simulink model "Buck_converter"  (R2015a)
settings: Solver=ode45  StartTime=0.0  StopTime=1.0  MaxStep=0.000001  MinStep=0.0000001  RelTol=1e-3
libraries: powerlib x12, simulink x1
settings Model: Creator=hp  LastModifiedBy=hp

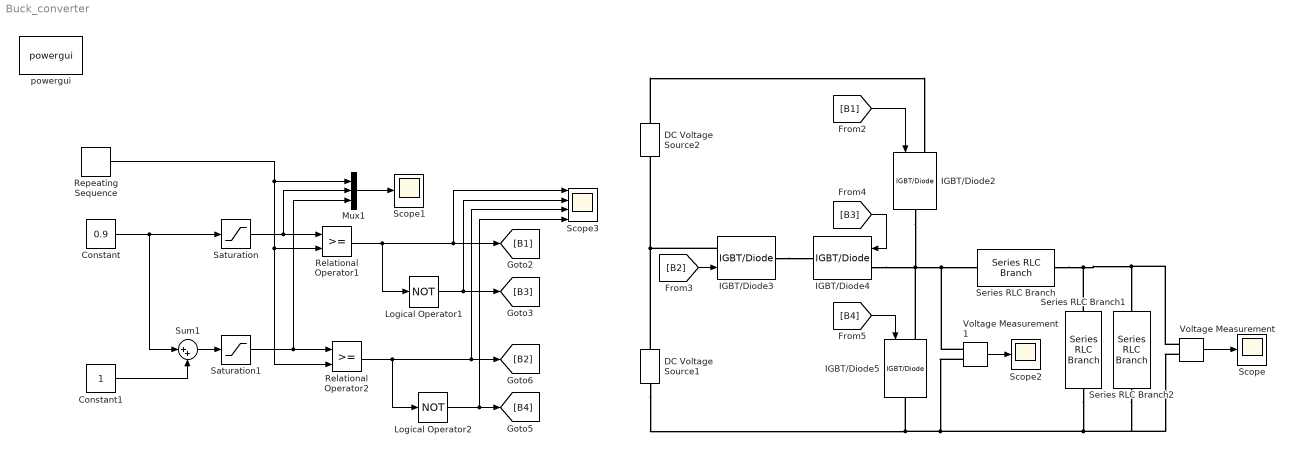
== system Buck_converter ==
  Constant : Constant  Value=0.9
  Constant1 : Constant
  DC Voltage Source1 : powerlib/Electrical Sources/DC Voltage Source  Amplitude=100  Measurements=None
  DC Voltage Source2 : powerlib/Electrical Sources/DC Voltage Source  Amplitude=100  Measurements=None
  IGBT/Diode{2..5} (4 alike) : powerlib/Power Electronics/IGBT//Diode  Ron=1e-3  Rs=1e5  Cs=inf  Measurements=off
  Logical Operator1 : Logic  Operator=NOT  Inputs=1  AllPortsSameDT=off  OutDataTypeStr=boolean
  Logical Operator2 : Logic  Operator=NOT  Inputs=1  AllPortsSameDT=off  OutDataTypeStr=boolean
  Mux1 : Mux  Inputs=3
  Relational Operator1 : RelationalOperator  OutDataTypeStr=boolean
  Relational Operator2 : RelationalOperator  OutDataTypeStr=boolean
  Repeating Sequence : simulink/Sources/Repeating Sequence  rep_seq_t=[0 0.5 1]/5000  rep_seq_y=[0 1 0]
  Saturation : Saturate  UpperLimit=1.0  LowerLimit=0
  Saturation1 : Saturate  UpperLimit=1.0  LowerLimit=0
  Scope : Scope
      settings: YMin=-10  YMax=220
  Scope1 : Scope
  Scope2 : Scope
      settings: YMin=2.99755e-06  YMax=2.99755e-06  SaveName=ScopeData2
  Scope3 : Scope  NumInputPorts=4
      settings: YMin=-5~-5~-5~-5  YMax=5~5~5~5  SaveName=ScopeData3
  Series RLC Branch : powerlib/Elements/Series RLC Branch  LConnTagsString=__new0  RConnTagsString=__new0  BranchType=L  Resistance=1  Inductance=1e-3  SetiL0=off  InitialCurrent=0  Capacitance=1e-6  Setx0=off  InitialVoltage=0  Measurements=None
  Series RLC Branch1 : powerlib/Elements/Series RLC Branch  LConnTagsString=__new0  RConnTagsString=__new0  BranchType=C  Resistance=1  Inductance=1e-3  SetiL0=off  InitialCurrent=0  Capacitance=1000e-6  Setx0=off  InitialVoltage=0  Measurements=None
  Series RLC Branch2 : powerlib/Elements/Series RLC Branch  LConnTagsString=__new0  RConnTagsString=__new0  BranchType=R  Resistance=1  Inductance=1e-3  SetiL0=off  InitialCurrent=0  Capacitance=1000e-6  Setx0=off  InitialVoltage=0  Measurements=None
  Sum1 : Sum  Inputs=|++
  Voltage Measurement : powerlib/Measurements/Voltage Measurement  PhasorSimulation=off  OutputType=Complex  PSBequivalent=0
  Voltage Measurement1 : powerlib/Measurements/Voltage Measurement  PhasorSimulation=off  OutputType=Complex  PSBequivalent=0
  powergui : powerlib/powergui  Priority=1  SimulationMode=Continuous  SolverType=Tustin/Backward Euler (TBE)  SampleTime=50e-6  frequency=60  SPID=off  DisableSnubberDevices=off  DisableRonSwitches=off  DisableVfSwitches=off  SwTol=0  DisplayEquations=off  Interpol=off  methode=off  Ts=100  FunctionMessages=off  echomessages=off  HookPort=off  EnableUseOfTLC=off  x0status=blocks  frequencyindice=0  Pbase=100e6  ErrMax=1e-4  Iterations=50  UnitsV=kV  UnitsW=MW  buscounter=0  RestoreLinks=warning  ResistiveCurrentMeasurement=off  Frange=[0:2:500]  Ylog=off  Xlog=on  ShowGrid=off  save=off  variable=ZData  structure=ScopeData3  ZoomFFT=on  StartTime=0.04  cycles=5  DisplayStyle=2  fundamental=50  FreqAxis=off  MaxFrequency=100000  frequencyindicesteady=1  RmsSteady=1  display=off
  wires:
  [B1] -> IGBT/Diode2/1
  [B4] -> IGBT/Diode5/1
  Relational Operator1/1 -> Logical Operator1/1, Scope3/1, [B1]
  Logical Operator1/1 -> Scope3/2, [B3]
  Constant/1 -> Sum1/1, Saturation/1
  Relational Operator2/1 -> Scope3/3, [B2], Logical Operator2/1
  Logical Operator2/1 -> Scope3/4, [B4]
  Saturation1/1 -> Mux1/3, Relational Operator2/1
  Sum1/1 -> Saturation1/1
  Constant1/1 -> Sum1/2
  Repeating Sequence/1 -> Mux1/1, Relational Operator2/2, Relational Operator1/2
  Mux1/1 -> Scope1/1
  Saturation/1 -> Mux1/2, Relational Operator1/1
  Voltage Measurement/1 -> Scope/1
  Voltage Measurement1/1 -> Scope2/1
  [B3] -> IGBT/Diode4/1
  [B2] -> IGBT/Diode3/1
  connections:
  DC Voltage Source1/RConn1 -- IGBT/Diode3/LConn1 -- DC Voltage Source2/LConn1
  DC Voltage Source2/RConn1 -- IGBT/Diode2/LConn1
  DC Voltage Source1/LConn1 -- Voltage Measurement/LConn2 -- Series RLC Branch2/RConn1 -- Series RLC Branch1/RConn1 -- Voltage Measurement1/LConn2 -- IGBT/Diode5/RConn1
  Series RLC Branch/RConn1 -- Voltage Measurement/LConn1 -- Series RLC Branch2/LConn1 -- Series RLC Branch1/LConn1
  IGBT/Diode3/RConn1 -- IGBT/Diode4/RConn1
  IGBT/Diode4/LConn1 -- IGBT/Diode2/RConn1 -- IGBT/Diode5/LConn1 -- Voltage Measurement1/LConn1 -- Series RLC Branch/LConn1
